simulink model "CtrPlatform"  (Simulink 7.9)
settings: Solver=ode3  StartTime=0.0  StopTime=8  FixedStep=Ts  RelTol=1e-3
InitFcn:
  | eval('CtrPlatformCfg')
StopFcn:
  | eval('CtrPlotTrj')
values from neighbouring files (symbols this model uses):
  A = [a1 a2 a3 a4 a5 a6]/180*pi    [Config.m]    (also in CtrPlatformCfg.m)
  a2 = 0    [Config.m]    (also in CtrPlatformCfg.m)
  a3 = 0    [Config.m]    (also in CtrPlatformCfg.m)
  a4 = 0    [Config.m]    (also in CtrPlatformCfg.m)
  a5 = 90    [Config.m]    (also in CtrPlatformCfg.m)
  a6 = 0    [Config.m]    (also in CtrPlatformCfg.m)
  Cen = Cen(:)'    [Config.m]    (also in CtrPlatformCfg.m; DynEulerTest.m = Cen'; EfDynCAD.m = [cen1,cen2,cen3,cen4,cen5,cen6]')
  CurPulseFreq = 0.25*2*pi    (= 1.57079632679)    [Config.m]    (also in CtrPlatformCfg.m)
  Deg2Rad = pi/180    (= 0.0174532925199)    [Config.m]    (also in CtrPlatformCfg.m)
  DisturbSelect = 2    [Config.m]    (also in CtrPlatformCfg.m)
  DynTrjMode = 3    [Config.m]    (also in CtrPlatformCfg.m = 1)
  FbDisturbSelect = 2    [Config.m]    (also in CtrPlatformCfg.m)
  freq = tvel/radius    (= 1)    [Config.m]    (also in CtrPlatformCfg.m)
  FrictionSelect = 2    [CtrPlatformCfg.m]
  Gravity = 9.8    [Config.m]    (also in CtrPlatformCfg.m)
  Ie1 = in1(:)'    [Config.m]    (also in CtrPlatformCfg.m; DynEulerTest.m = in1(:); EfDynCAD.m = in1(:))
  Ie2 = in2(:)'    [Config.m]    (also in CtrPlatformCfg.m; DynEulerTest.m = in2(:); EfDynCAD.m = in2(:))
  Ie3 = in3(:)'    [Config.m]    (also in CtrPlatformCfg.m; DynEulerTest.m = in3(:); EfDynCAD.m = in3(:))
  Ie4 = in4(:)'    [Config.m]    (also in CtrPlatformCfg.m; DynEulerTest.m = in4(:); EfDynCAD.m = in4(:))
  Ie5 = in5(:)'    [Config.m]    (also in CtrPlatformCfg.m; DynEulerTest.m = in5(:); EfDynCAD.m = in5(:))
  Ie6 = in6(:)'    [Config.m]    (also in CtrPlatformCfg.m; DynEulerTest.m = in6(:); EfDynCAD.m = in6(:))
  in1 = [5.2954 -0.2565 -0.6366;-0.2565 4.7000 0.2830;-0.6366 0.2829 5.8635]    [Config.m]    (also in CtrPlatformCfg.m; DynEulerTest.m; EfDynCAD.m = [0.54  -0.01 0.23)
  in2 = [5.8840 0.0072 0.0135;0.0072 6.0178 -0.1907;0.0135 -0.1907 0.3374]    [Config.m]    (also in CtrPlatformCfg.m; DynEulerTest.m; EfDynCAD.m = (R_x*R_z)*in2*(R_x*R_z)')
  in3 = [1.8201 -0.2274 -0.3112;-0.2274 2.2537 -0.1441;-0.3112 -0.1441 1.9485]    [Config.m]    (also in CtrPlatformCfg.m; DynEulerTest.m; EfDynCAD.m = (R_x*R_z)*in3*(R_x*R_z)')
  in4 = [0.0607 -0.0922 0;-0.0922 1.4493 0;0 0 1.4620]    [Config.m]    (also in CtrPlatformCfg.m; DynEulerTest.m = [0.0607 -0.0922 0;-0.0922 1.4493 0;0 0,1.4620]; EfDynCAD.m = (R_y*Rz)*in4*(R_y*Rz)')
  in5 = [0.0191 0.0032 0;0.0032 0.0228 0;0 0 0.0291]    [Config.m]    (also in CtrPlatformCfg.m; DynEulerTest.m; EfDynCAD.m = (R_x*R_y)*in5*(R_x*R_y)')
  in6 = [0.0012 0 0;0 0.0007 0;0 0 0.0007]    [Config.m]    (also in CtrPlatformCfg.m; DynEulerTest.m; EfDynCAD.m = (R_y*Rz)*in6*(R_y*Rz)')
  init_Endx = gd_init(1,4)    [Config.m]    (also in CtrPlatformCfg.m)
  init_Endy = gd_init(2,4)    [Config.m]    (also in CtrPlatformCfg.m)
  init_Endz = gd_init(3,4)    [Config.m]    (also in CtrPlatformCfg.m)
  init_Rot = gd_init(1:3,1:3)    [Config.m]    (also in CtrPlatformCfg.m)
  JntOffset1 = A(1)    [Config.m]    (also in CtrPlatformCfg.m)
  JntOffset2 = A(2)    [Config.m]    (also in CtrPlatformCfg.m)
  JntOffset3 = A(3)    [Config.m]    (also in CtrPlatformCfg.m)
  JntOffset4 = A(4)    [Config.m]    (also in CtrPlatformCfg.m)
  JntOffset5 = A(5)    [Config.m]    (also in CtrPlatformCfg.m)
  JntOffset6 = A(6)    [Config.m]    (also in CtrPlatformCfg.m)
  L = [l1 l2 l3 l4 l5 l6 l7 l8 l9]    [Config.m]    (also in CtrPlatformCfg.m)
  LinePTs2RadpS = 2*pi/(EncRes*Ts)./Gear    [Config.m]    (also in CtrPlatformCfg.m)
  LinePTs2Rpm = 60/(EncRes*Ts)    (= 7.32421875)    [Config.m]    (also in CtrPlatformCfg.m)
  Ma = [ma1 ma2 ma3 ma4 ma5 ma6]    [Config.m]    (also in CtrPlatformCfg.m; DynEulerTest.m = [ma1; ma2; ma3; ma4; ma5; ma6]; EfDynCAD.m = [ma1 ma2 ma3 ma4 ma5 ma6]')
  ma1 = 170.31    [Config.m]    (also in CtrPlatformCfg.m; DynEulerTest.m; EfDynCAD.m = 77.75)
  ma2 = 63.74    [Config.m]    (also in CtrPlatformCfg.m; DynEulerTest.m; EfDynCAD.m = 32.31)
  ma3 = 98.98    [Config.m]    (also in CtrPlatformCfg.m; DynEulerTest.m; EfDynCAD.m = 18.61)
  ma4 = 24.46    [Config.m]    (also in CtrPlatformCfg.m; DynEulerTest.m; EfDynCAD.m = 15.65)
  ma5 = 5.24    [Config.m]    (also in CtrPlatformCfg.m; DynEulerTest.m; EfDynCAD.m = 3.32)
  ma6 = 0.6    [Config.m]    (also in CtrPlatformCfg.m; DynEulerTest.m; EfDynCAD.m)
  PosPulseEnable = 1    [Config.m]    (also in CtrPlatformCfg.m)
  PosVelPulseGain = 500    [Config.m]    (also in CtrPlatformCfg.m)
  Rad2Line = Gear*EncRes/(2*pi)    [Config.m]    (also in CtrPlatformCfg.m)
  Rpm2LinePTs = EncRes*Ts/60    (= 0.136533333333)    [Config.m]    (also in CtrPlatformCfg.m)
  TrajSwitch = 1    [Config.m]    (also in CtrPlatformCfg.m)
  Trq2Cur = Trq2Cur./Cur2Trq    [Config.m]    (also in CtrPlatformCfg.m)
  Ts = 1/FrHz    (= 0.00025)    [Config.m]    (also in CtrPlatformCfg.m)
  Ts_Dyn = Ts    (= 0.00025)    [Config.m]    (also in CtrPlatformCfg.m)
  tvel = 120    [Config.m]    (also in CtrPlatformCfg.m)
  VelLpAxisNum = 1    [Config.m]    (also in CtrPlatformCfg.m)
  VelPulseEnable = 0    [Config.m]    (also in CtrPlatformCfg.m)
  VelPulseGain = 500    [Config.m]    (also in CtrPlatformCfg.m)
  Volt2Trq = Volt2Trq./Trq2Cur    [Config.m]    (also in CtrPlatformCfg.m)
undefined symbols (not defined in the file or in its folder): a1, DiscIntNeverNeededParam, RobotAxis
libraries: simulink x85, mblibv1 x35, powerlib_extras x25, commnoisgen2 x2
(part 1 of 5)
settings Model: Creator=DAI Dan  LastModifiedBy=Administrator
settings DebuggingCC: FcnCallInpInsideContextMsg=Use local settings
settings GRTTargetCC: CombineOutputUpdateFcns=off  GRTInterface=on
settings ConfigurationSet: Description=SimMechanics 2G

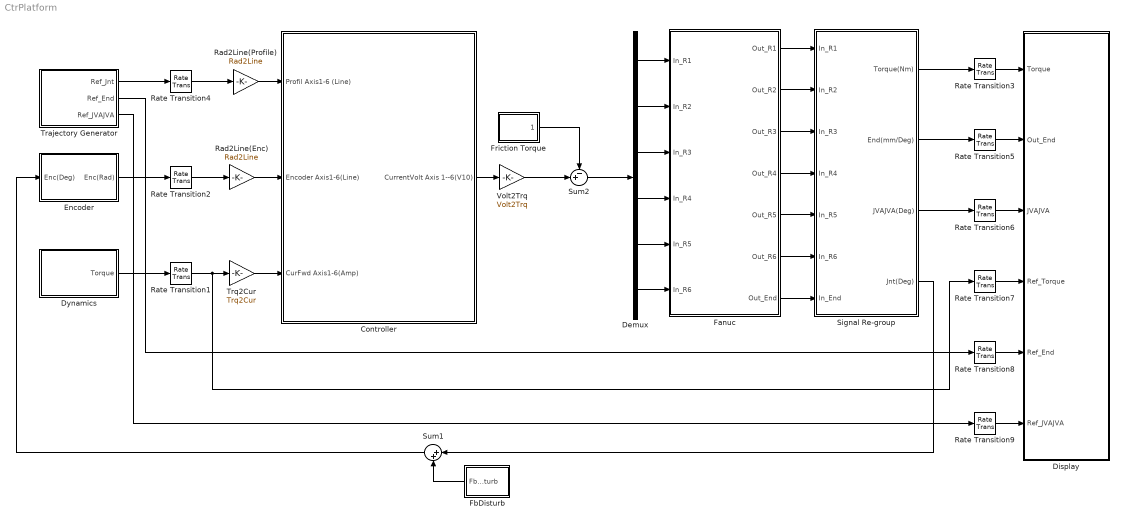
== system CtrPlatform ==
  Controller : Subsystem
  Demux : Demux  Outputs=6
  Display : Subsystem
  Dynamics : Subsystem
  Encoder : Subsystem
  Fanuc : Subsystem
  FbDisturb : Subsystem
  Friction Torque : Subsystem
  Rad2Line(Enc) : Gain  Gain=Rad2Line
  Rad2Line(Profile) : Gain  Gain=Rad2Line
  Rate Transition{1..9} (9 alike) : RateTransition  OutPortSampleTime=Ts
  Signal Re-group : Subsystem
  Sum1 : Sum  Inputs=|++
  Sum2 : Sum  Inputs=-+|
  Trajectory Generator : Subsystem
  Trq2Cur : Gain  Gain=Trq2Cur
  Volt2Trq : Gain  Gain=Volt2Trq  SampleTime=Ts
  wires:
  Trq2Cur/1 -> Controller/3(CurFwd Axis1-6(Amp))
  Rad2Line(Profile)/1 -> Controller/1(Profil Axis1-6 (Line))
  Rad2Line(Enc)/1 -> Controller/2(Encoder Axis1-6(Line))
  Controller/1(CurrentVolt Axis 1--6(V10)) -> Volt2Trq/1
  Rate Transition4/1 -> Rad2Line(Profile)/1
  Rate Transition1/1 -> Trq2Cur/1, Rate Transition7/1
  Rate Transition2/1 -> Rad2Line(Enc)/1
  FbDisturb/1(FbDisturb) -> Sum1/2
  Demux/1 -> Fanuc/1(In_R1)
  Demux/2 -> Fanuc/2(In_R2)
  Demux/3 -> Fanuc/3(In_R3)
  Demux/4 -> Fanuc/4(In_R4)
  Demux/5 -> Fanuc/5(In_R5)
  Demux/6 -> Fanuc/6(In_R6)
  Fanuc/1(Out_R1) -> Signal Re-group/1(In_R1)
  Fanuc/2(Out_R2) -> Signal Re-group/2(In_R2)
  Fanuc/3(Out_R3) -> Signal Re-group/3(In_R3)
  Fanuc/4(Out_R4) -> Signal Re-group/4(In_R4)
  Fanuc/5(Out_R5) -> Signal Re-group/5(In_R5)
  Fanuc/6(Out_R6) -> Signal Re-group/6(In_R6)
  Fanuc/7(Out_End) -> Signal Re-group/7(In_End)
  Signal Re-group/1(Torque(Nm)) -> Rate Transition3/1
  Signal Re-group/2(End(mm/Deg)) -> Rate Transition5/1
  Signal Re-group/3(JVAJVA(Deg)) -> Rate Transition6/1
  Rate Transition3/1 -> Display/1(Torque)
  Rate Transition5/1 -> Display/2(Out_End)
  Rate Transition6/1 -> Display/3(JVAJVA)
  Rate Transition7/1 -> Display/4(Ref_Torque)
  Rate Transition8/1 -> Display/5(Ref_End)
  Rate Transition9/1 -> Display/6(Ref_JVAJVA)
  Signal Re-group/4(Jnt(Deg)) -> Sum1/1
  Sum2/1 -> Demux/1
  Volt2Trq/1 -> Sum2/2
  Friction Torque/1(Friction) -> Sum2/1
  Trajectory Generator/1(Ref_Jnt) -> Rate Transition4/1
  Dynamics/1(Torque) -> Rate Transition1/1
  Encoder/1(Enc(Rad)) -> Rate Transition2/1
  Sum1/1 -> Encoder/1(Enc(Deg))
  Trajectory Generator/2(Ref_End) -> Rate Transition8/1
  Trajectory Generator/3(Ref_JVAJVA) -> Rate Transition9/1

== system CtrPlatform/Controller ==
  Profil Axis1-6 (Line) : Inport
  Encoder Axis1-6(Line) : Inport  Port=2
  CurFwd Axis1-6(Amp) : Inport  Port=3
  Chech Axis Error Flag : Logic  Inputs=6  AllPortsSameDT=off  OutDataTypeStr=boolean
  Controller Axis 1 : Subsystem  mask{RobotAxis=RobotAxis(1), Ts=Ts}
      mask prompts: RobotAxis "Robot Axis Controller Parameter"; Ts "Sample Time"
      mask init:
      | %% Source and Control Loop Selection
      | PosSourceSelect=RobotAxis.PosSourceSelect;
      | VelSourceSelect=RobotAxis.VelSourceSelect;
      | CurSourceSelect=RobotAxis.CurSourceSelect;
      | FilterSelect=RobotAxis.FilterSelect;
      | FwdSelect=RobotAxis.FwdSelect;
      | AxisNO=RobotAxis.AxisNO;
      | 
      | %% Controller Parameter
      | Kpp=RobotAxis.Kpp; % Kp for position loop
      | Kpi=RobotAxis.Kpi; 
      | Kpd=RobotAxis.Kpd;
      | VelLimit=RobotAxis.VelLimit;
      | 
      | Kvp=RobotAxis.Kvp; % Kp for velocity loop
      | Kvi=RobotAxis.Kvi;
      | Kvd=RobotAxis.Kvd;
      | CurLimit = RobotAxis.CurLimit;
      | 
      | Cur2Volt=RobotAxis.Cur2Volt;
      | 
      | %% Feedforward Param
      | VelFwdGain=RobotAxis.VelFwdGain;
      | CurFwdGain=RobotAxis.CurFwdGain;
      | 
      | %% Protection
      | VelErrorCheckLimit=RobotAxis.VelErrorCheckLimit;
      | PosErrorCheckLimit=RobotAxis.PosErrorCheckLimit;
      | 
      | %% Initial Positon (Line)
      | InitialPos=RobotAxis.InitialPos;
  Controller Axis 2 : Subsystem  mask{RobotAxis=RobotAxis(2), Ts=Ts}
      mask prompts: RobotAxis "Robot Axis Controller Parameter"; Ts "Sample Time"
      mask init: same as CtrPlatform/Controller/Controller Axis 1
  Controller Axis 3 : Subsystem  mask{RobotAxis=RobotAxis(3), Ts=Ts}
      mask prompts: RobotAxis "Robot Axis Controller Parameter"; Ts "Sample Time"
      mask init: same as CtrPlatform/Controller/Controller Axis 1
  Controller Axis 4 : Subsystem  mask{RobotAxis=RobotAxis(4), Ts=Ts}
      mask prompts: RobotAxis "Robot Axis Controller Parameter"; Ts "Sample Time"
      mask init: same as CtrPlatform/Controller/Controller Axis 1
  Controller Axis 5 : Subsystem  mask{RobotAxis=RobotAxis(5), Ts=Ts}
      mask prompts: RobotAxis "Robot Axis Controller Parameter"; Ts "Sample Time"
      mask init: same as CtrPlatform/Controller/Controller Axis 1
  Controller Axis 6 : Subsystem  mask{RobotAxis=RobotAxis(6), Ts=Ts}
      mask prompts: RobotAxis "Robot Axis Controller Parameter"; Ts "Sample Time"
      mask init: same as CtrPlatform/Controller/Controller Axis 1
  Disturb : Subsystem
  ErrDisplay : Scope
      settings: SaveName=ScopeData12
  Integer Delay : Delay  DelayLength=1  InitialCondition=A'.*Rad2Line  SampleTime=Ts
  Mux : Mux  Inputs=6
  Source Model : Subsystem
  Sum2 : Sum  Inputs=++|
  CurrentVolt Axis 1--6(V10) : Outport
  wires:
  Chech Axis Error Flag/1 -> ErrDisplay/1
  Profil Axis1-6 (Line)/1 -> Controller Axis 1/1(Prof), Controller Axis 2/1(Prof), Controller Axis 5/1(Prof), Controller Axis 6/1(Prof), Controller Axis 4/1(Prof), Controller Axis 3/1(Prof)
  Encoder Axis1-6(Line)/1 -> Integer Delay/1
  CurFwd Axis1-6(Amp)/1 -> Controller Axis 1/3(CurFwd), Controller Axis 2/3(CurFwd), Controller Axis 3/3(CurFwd), Controller Axis 5/3(CurFwd), Controller Axis 6/3(CurFwd), Controller Axis 4/3(CurFwd)
  Controller Axis 1/1(CurrentVolt(V10)) -> Mux/1  "Volt Axis1"
  Controller Axis 2/1(CurrentVolt(V10)) -> Mux/2
  Controller Axis 3/1(CurrentVolt(V10)) -> Mux/3
  Controller Axis 4/1(CurrentVolt(V10)) -> Mux/4
  Controller Axis 5/1(CurrentVolt(V10)) -> Mux/5
  Controller Axis 6/1(CurrentVolt(V10)) -> Mux/6
  Controller Axis 1/2(ErrFlag) -> Chech Axis Error Flag/1  "Error Axis1"
  Controller Axis 2/2(ErrFlag) -> Chech Axis Error Flag/2
  Controller Axis 3/2(ErrFlag) -> Chech Axis Error Flag/3
  Controller Axis 4/2(ErrFlag) -> Chech Axis Error Flag/4
  Controller Axis 5/2(ErrFlag) -> Chech Axis Error Flag/5
  Controller Axis 6/2(ErrFlag) -> Chech Axis Error Flag/6
  Integer Delay/1 -> Controller Axis 1/2(Enc), Controller Axis 2/2(Enc), Controller Axis 5/2(Enc), Controller Axis 6/2(Enc), Controller Axis 4/2(Enc), Controller Axis 3/2(Enc)
  Mux/1 -> Sum2/2
  Sum2/1 -> CurrentVolt Axis 1--6(V10)/1
  Disturb/1(Disturb) -> Sum2/1

== system CtrPlatform/Display ==
  Torque : Inport
  Out_End : Inport  Port=2
  JVAJVA : Inport  Port=3
  Ref_Torque : Inport  Port=4
  Ref_End : Inport  Port=5
  Ref_JVAJVA : Inport  Port=6
  EndTrjDisplay : Subsystem
  JntVelAccDisplay : Subsystem
  TorqueDisplay : Subsystem
  wires:
  Torque/1 -> TorqueDisplay/1(Torque)
  Ref_Torque/1 -> TorqueDisplay/2(Ref_Torque)
  JVAJVA/1 -> JntVelAccDisplay/1(JointVelAcc)
  Ref_JVAJVA/1 -> JntVelAccDisplay/2(Ref_JntVelAcc)
  Out_End/1 -> EndTrjDisplay/1(End)
  Ref_End/1 -> EndTrjDisplay/2(RefEnd)

== system CtrPlatform/Dynamics ==
  C*Omega : MATLAB Function  TreatAsAtomicUnit=on
  C_Omega Display : Subsystem
  M*Acc : MATLAB Function  TreatAsAtomicUnit=on
  M_Acc Display : Subsystem
  N : MATLAB Function  TreatAsAtomicUnit=on
  N Display : Subsystem
  Rate Transition1 : RateTransition  OutPortSampleTime=Ts_Dyn
  Rate Transition2 : RateTransition  OutPortSampleTime=Ts_Dyn
  Rate Transition3 : RateTransition  OutPortSampleTime=Ts_Dyn
  Sum : Sum  Inputs=+++
  Terminator : Terminator
  Terminator1 : Terminator
  Terminator2 : Terminator
  Torque Display : Subsystem
  TrjSource : Subsystem
  Torque : Outport
  wires:
  M*Acc/1(M_Acc) -> Sum/1, M_Acc Display/1(M_Acc)
  C*Omega/1(C_Omega) -> Sum/3, C_Omega Display/1(C_Omega)
  Sum/1 -> Torque/1, Torque Display/1(Torque)
  N/1(N) -> Sum/2, N Display/1(N)
  [RobotEncPos] -> Rate Transition1/1
  [RobotEncVel] -> Rate Transition2/1
  [RobotEncAcc] -> Rate Transition3/1
  Rate Transition1/1 -> Terminator/1
  Rate Transition2/1 -> Terminator1/1
  Rate Transition3/1 -> Terminator2/1
  TrjSource/1(RefJntPos(Rad)) -> M*Acc/2(EnTheta), N/1(EnTheta), C*Omega/2(EnTheta)
  TrjSource/2(RefJntVel(Rad/s)) -> C*Omega/1(RefOmega), C*Omega/3(EnOmega)
  TrjSource/3(RefJntAcc(Rad/s2)) -> M*Acc/1(RefAcc)

== system CtrPlatform/Encoder ==
  Enc(Deg) : Inport
  Deg2Rad : Gain  Gain=Deg2Rad
  Demux1 : Demux  Outputs=6
  Dir{1..6} (6 alike) : Gain
  Mux : Mux  Inputs=6
  Enc(Rad) : Outport
  wires:
  Enc(Deg)/1 -> Deg2Rad/1
  Dir1/1 -> Mux/1
  Mux/1 -> Enc(Rad)/1
  Deg2Rad/1 -> Demux1/1
  Dir2/1 -> Mux/2
  Dir3/1 -> Mux/3
  Demux1/6 -> Dir6/1
  Dir6/1 -> Mux/6
  Dir5/1 -> Mux/5
  Dir4/1 -> Mux/4
  Demux1/5 -> Dir5/1
  Demux1/4 -> Dir4/1
  Demux1/3 -> Dir3/1
  Demux1/2 -> Dir2/1
  Demux1/1 -> Dir1/1

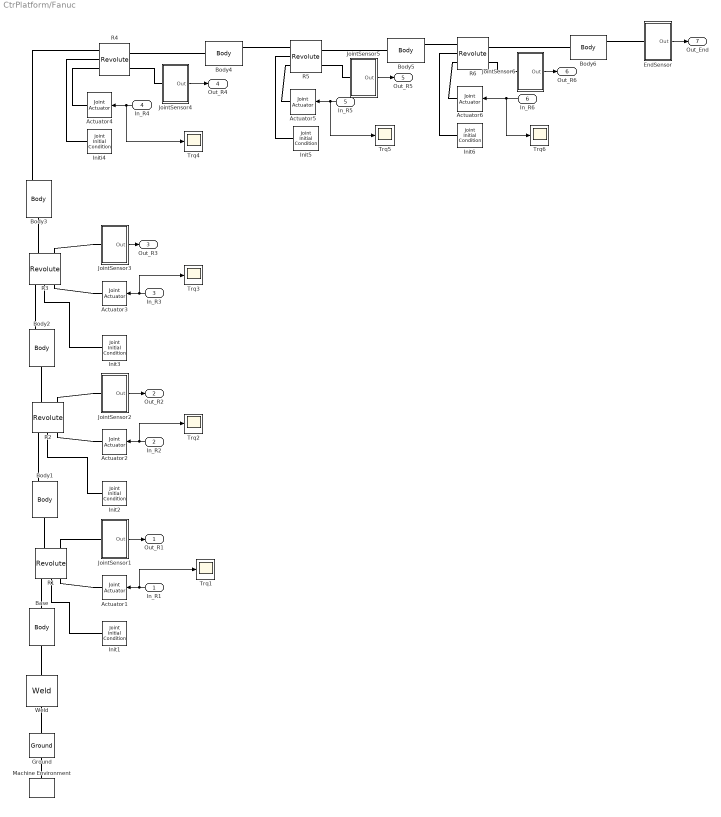
== system CtrPlatform/Fanuc ==
  In_R1 : Inport
  In_R2 : Inport  Port=2
  In_R3 : Inport  Port=3
  In_R4 : Inport  Port=4
  In_R5 : Inport  Port=5
  In_R6 : Inport  Port=6
  " EndSensor" : Subsystem
  Actuator{1..6} (6 alike) : mblibv1/Sensors &  Actuators/Joint Actuator  UpdateFromCAD=off  PhysicalDomain=Mechanical  PortType=blob  ActuationStyle=Force  AngleUnits=rad  ArcVelocityUnits=rad/s  ArcAccelerationUnits=rad/s^2  CoordPositionUnits=m  VelocityUnits=m/s  AccelerationUnits=m/s^2  ForceUnits=N  TorqueUnits=N*m  ActiveIO=on  Width=1  DialogClass=MechanicalActuatorBlock  Primitive=R1  ReferenceFrame=Absolute (World)
  Base : mblibv1/Bodies/Body  LConnTagsString=CS1  RConnTagsString=CS2  UpdateFromCAD=on  DialogClass=MechanicalBodyBlock  Mass=133.95  MassUnits=kg  InertiaUnits=kg*m^2  Inertia=[3.0977 0.0155 -0.0939;0.0155 3.3580 0.0061;-0.0939 0.0061 5.1969]  Shape=Cylinder  ShapeDims=[1 1]  ShapeUnits=m  ShapeUse=false  Density=1  DensityUnits=kg/m^3  DensityUse=false  GraphicsMode=GFXFILE  GraphicsFileName=M-710iC50 M-710iC70 - M-710iC50 M-710iC70 base-1.STL  BodyColorSelMode=COLORPALETTE  BodyColor=[0.25098 0.25098 0.25098]  AttachedToCS=CS1  CG=Right$CG$[-0.0437 -0.0026 0.1059]$WORLD$WORLD$m$[1 0 0;0 1 0;0 0 1]$3x3 Transform$rad$WORLD$false$none  WorkingFrames=Left$CS1$[0 0 0]$WORLD$WORLD$m$[1 0 0;0 1 0;0 0 1]$3x3 Transform$rad$WORLD$true$none#Right$CS2$[0 0 0.266]$WORLD$WORLD$m$[1 0 0;0 1 0;0 0 1]$3x3 Transform$rad$WORLD$true$none  CGPos=[-0.0437 -0.0026 0.1059]  CGRot=[1 0 0;0 1 0;0 0 1]  CS0Pos=[]  CS0Rot=[]  CS1Pos=[0 0 0]  CS1Rot=[1 0 0;0 1 0;0 0 1]  CS2Pos=[0 0 0.266]  CS2Rot=[1 0 0;0 1 0;0 0 1]  CS3Pos=[]  CS3Rot=[]  CS4Pos=[]  CS4Rot=[]  CS5Pos=[]  CS5Rot=[]  CS6Pos=[]  CS6Rot=[]  CS7Pos=[]  CS7Rot=[]  CS8Pos=[]  CS8Rot=[]  CS9Pos=[]  CS9Rot=[]  CS10Pos=[]  CS10Rot=[]  CS11Pos=[]  CS11Rot=[]  CS12Pos=[]  CS12Rot=[]  CS13Pos=[]  CS13Rot=[]  CS14Pos=[]  CS14Rot=[]  CS15Pos=[]  CS15Rot=[]  CS16Pos=[]  CS16Rot=[]  CS17Pos=[]  CS17Rot=[]  CS18Pos=[]  CS18Rot=[]  CS19Pos=[]  CS19Rot=[]  CS20Pos=[]  CS20Rot=[]
  Body1 : mblibv1/Bodies/Body  LConnTagsString=CS2  RConnTagsString=CS3|CS4  UpdateFromCAD=on  DialogClass=MechanicalBodyBlock  Mass=ma1  MassUnits=kg  InertiaUnits=kg*m^2  Inertia=in1  Shape=Cylinder  ShapeDims=[1 1]  ShapeUnits=m  ShapeUse=false  Density=1  DensityUnits=kg/m^3  DensityUse=false  GraphicsMode=GFXFILE  GraphicsFileName=M-710iC50 M-710iC70 - M-710iC50 M-710iC70 axis1-1.STL  BodyColorSelMode=COLORPALETTE  BodyColor=[0.86667 0.86667 0.8902]  AttachedToCS=CS1  CG=Right$CG$cen1$WORLD$WORLD$m$[1 0 0;0 1 0;0 0 1]$3x3 Transform$rad$WORLD$false$none  WorkingFrames=Right$CS1$cen1_1$WORLD$WORLD$m$[1 0 0;0 1 0;0 0 1]$3x3 Transform$rad$WORLD$false$none#Left$CS2$cen1_2$WORLD$WORLD$m$[1 0 0;0 1 0;0 0 1]$3x3 Transform$rad$WORLD$true$none#Right$CS3$cen1_3$WORLD$WORLD$m$[1 0 0;0 1 0;0 0 1]$3x3 Transform$rad$WORLD$true$none#Right$CS4$cen1_4$WORLD$WORLD$m$[1 0 0;0 1 0;0 0 1]$3x3 Transform$rad$WORLD$true$none  CGPos=cen1  CGRot=[1 0 0;0 1 0;0 0 1]  CS0Pos=[]  CS0Rot=[]  CS1Pos=cen1_1  CS1Rot=[1 0 0;0 1 0;0 0 1]  CS2Pos=cen1_2  CS2Rot=[1 0 0;0 1 0;0 0 1]  CS3Pos=cen1_3  CS3Rot=[1 0 0;0 1 0;0 0 1]  CS4Pos=cen1_4  CS4Rot=[1 0 0;0 1 0;0 0 1]  CS5Pos=[]  CS5Rot=[]  CS6Pos=[]  CS6Rot=[]  CS7Pos=[]  CS7Rot=[]  CS8Pos=[]  CS8Rot=[]  CS9Pos=[]  CS9Rot=[]  CS10Pos=[]  CS10Rot=[]  CS11Pos=[]  CS11Rot=[]  CS12Pos=[]  CS12Rot=[]  CS13Pos=[]  CS13Rot=[]  CS14Pos=[]  CS14Rot=[]  CS15Pos=[]  CS15Rot=[]  CS16Pos=[]  CS16Rot=[]  CS17Pos=[]  CS17Rot=[]  CS18Pos=[]  CS18Rot=[]  CS19Pos=[]  CS19Rot=[]  CS20Pos=[]  CS20Rot=[]
  Body2 : mblibv1/Bodies/Body  LConnTagsString=CS2  RConnTagsString=CS3|CS4  UpdateFromCAD=on  DialogClass=MechanicalBodyBlock  Mass=ma2  MassUnits=kg  InertiaUnits=kg*m^2  Inertia=in2  Shape=Cylinder  ShapeDims=[1 1]  ShapeUnits=m  ShapeUse=false  Density=1  DensityUnits=kg/m^3  DensityUse=false  GraphicsMode=GFXFILE  GraphicsFileName=M-710iC50 M-710iC70 - M-710iC50 M-710iC70 axis2-1.STL  BodyColorSelMode=COLORPALETTE  BodyColor=[1 1 0]  AttachedToCS=CS1  CG=Right$CG$cen2$WORLD$WORLD$m$[1 0 0;0 1 0;0 0 1]$3x3 Transform$rad$WORLD$false$none  WorkingFrames=Right$CS1$cen2_1$WORLD$WORLD$m$[1 0 0;0 1 0;0 0 1]$3x3 Transform$rad$WORLD$false$none#Left$CS2$cen2_2$WORLD$WORLD$m$[1 0 0;0 1 0;0 0 1]$3x3 Transform$rad$WORLD$true$none#Right$CS3$cen2_3$WORLD$WORLD$m$[1 0 0;0 1 0;0 0 1]$3x3 Transform$rad$WORLD$true$none#Right$CS4$cen2_4$WORLD$WORLD$m$[1 0 0;0 1 0;0 0 1]$3x3 Transform$rad$WORLD$true$none  CGPos=cen2  CGRot=[1 0 0;0 1 0;0 0 1]  CS0Pos=[]  CS0Rot=[]  CS1Pos=cen2_1  CS1Rot=[1 0 0;0 1 0;0 0 1]  CS2Pos=cen2_2  CS2Rot=[1 0 0;0 1 0;0 0 1]  CS3Pos=cen2_3  CS3Rot=[1 0 0;0 1 0;0 0 1]  CS4Pos=cen2_4  CS4Rot=[1 0 0;0 1 0;0 0 1]  CS5Pos=[]  CS5Rot=[]  CS6Pos=[]  CS6Rot=[]  CS7Pos=[]  CS7Rot=[]  CS8Pos=[]  CS8Rot=[]  CS9Pos=[]  CS9Rot=[]  CS10Pos=[]  CS10Rot=[]  CS11Pos=[]  CS11Rot=[]  CS12Pos=[]  CS12Rot=[]  CS13Pos=[]  CS13Rot=[]  CS14Pos=[]  CS14Rot=[]  CS15Pos=[]  CS15Rot=[]  CS16Pos=[]  CS16Rot=[]  CS17Pos=[]  CS17Rot=[]  CS18Pos=[]  CS18Rot=[]  CS19Pos=[]  CS19Rot=[]  CS20Pos=[]  CS20Rot=[]
  Body3 : mblibv1/Bodies/Body  LConnTagsString=CS2  RConnTagsString=CS3|CS4  UpdateFromCAD=on  DialogClass=MechanicalBodyBlock  Mass=ma3  MassUnits=kg  InertiaUnits=kg*m^2  Inertia=in3  Shape=Cylinder  ShapeDims=[1 1]  ShapeUnits=m  ShapeUse=false  Density=1  DensityUnits=kg/m^3  DensityUse=false  GraphicsMode=GFXFILE  GraphicsFileName=M-710iC50 M-710iC70 - M-710iC50 M-710iC70 axis3-1.STL  BodyColorSelMode=COLORPALETTE  BodyColor=[1 1 0]  AttachedToCS=CS1  CG=Right$CG$cen3$WORLD$WORLD$m$[1 0 0;0 1 0;0 0 1]$3x3 Transform$rad$WORLD$false$none  WorkingFrames=Right$CS1$cen3_1$WORLD$WORLD$m$[1 0 0;0 1 0;0 0 1]$3x3 Transform$rad$WORLD$false$none#Left$CS2$cen3_2$WORLD$WORLD$m$[1 0 0;0 1 0;0 0 1]$3x3 Transform$rad$WORLD$true$none#Right$CS3$cen3_3$WORLD$WORLD$m$[1 0 0;0 1 0;0 0 1]$3x3 Transform$rad$WORLD$true$none#Right$CS4$cen3_4$WORLD$WORLD$m$[1 0 0;0 1 0;0 0 1]$3x3 Transform$rad$WORLD$true$none  CGPos=cen3  CGRot=[1 0 0;0 1 0;0 0 1]  CS0Pos=[]  CS0Rot=[]  CS1Pos=cen3_1  CS1Rot=[1 0 0;0 1 0;0 0 1]  CS2Pos=cen3_2  CS2Rot=[1 0 0;0 1 0;0 0 1]  CS3Pos=cen3_3  CS3Rot=[1 0 0;0 1 0;0 0 1]  CS4Pos=cen3_4  CS4Rot=[1 0 0;0 1 0;0 0 1]  CS5Pos=[]  CS5Rot=[]  CS6Pos=[]  CS6Rot=[]  CS7Pos=[]  CS7Rot=[]  CS8Pos=[]  CS8Rot=[]  CS9Pos=[]  CS9Rot=[]  CS10Pos=[]  CS10Rot=[]  CS11Pos=[]  CS11Rot=[]  CS12Pos=[]  CS12Rot=[]  CS13Pos=[]  CS13Rot=[]  CS14Pos=[]  CS14Rot=[]  CS15Pos=[]  CS15Rot=[]  CS16Pos=[]  CS16Rot=[]  CS17Pos=[]  CS17Rot=[]  CS18Pos=[]  CS18Rot=[]  CS19Pos=[]  CS19Rot=[]  CS20Pos=[]  CS20Rot=[]
  Body4 : mblibv1/Bodies/Body  LConnTagsString=CS2  RConnTagsString=CS3|CS4  UpdateFromCAD=on  DialogClass=MechanicalBodyBlock  Mass=ma4  MassUnits=kg  InertiaUnits=kg*m^2  Inertia=in4  Shape=Cylinder  ShapeDims=[1 1]  ShapeUnits=m  ShapeUse=false  Density=1  DensityUnits=kg/m^3  DensityUse=false  GraphicsMode=GFXFILE  GraphicsFileName=M-710iC50 M-710iC70 - M-710iC50 M-710iC70 axis4-1.STL  BodyColorSelMode=COLORPALETTE  BodyColor=[1 1 0]  AttachedToCS=CS1  CG=Right$CG$cen4$WORLD$WORLD$m$[1 0 0;0 0 1;0 -1 0]$3x3 Transform$rad$WORLD$false$none  WorkingFrames=Right$CS1$cen4_1$WORLD$WORLD$m$[1 0 0;0 0 1;0 -1 0]$3x3 Transform$rad$WORLD$false$none#Left$CS2$cen4_2$WORLD$WORLD$m$[1 0 0;0 1 0;0 0 1]$3x3 Transform$rad$WORLD$true$none#Right$CS3$cen4_3$WORLD$WORLD$m$[1 0 0;0 1 0;0 0 1]$3x3 Transform$rad$WORLD$true$none#Right$CS4$cen4_4$WORLD$WORLD$m$[1 0 0;0 1 0;0 0 1]$3x3 Transform$rad$WORLD$true$none  CGPos=cen4  CGRot=[1 0 0;0 0 1;0 -1 0]  CS0Pos=[]  CS0Rot=[]  CS1Pos=cen4_1  CS1Rot=[1 0 0;0 0 1;0 -1 0]  CS2Pos=cen4_2  CS2Rot=[1 0 0;0 1 0;0 0 1]  CS3Pos=cen4_3  CS3Rot=[1 0 0;0 1 0;0 0 1]  CS4Pos=cen4_4  CS4Rot=[1 0 0;0 1 0;0 0 1]  CS5Pos=[]  CS5Rot=[]  CS6Pos=[]  CS6Rot=[]  CS7Pos=[]  CS7Rot=[]  CS8Pos=[]  CS8Rot=[]  CS9Pos=[]  CS9Rot=[]  CS10Pos=[]  CS10Rot=[]  CS11Pos=[]  CS11Rot=[]  CS12Pos=[]  CS12Rot=[]  CS13Pos=[]  CS13Rot=[]  CS14Pos=[]  CS14Rot=[]  CS15Pos=[]  CS15Rot=[]  CS16Pos=[]  CS16Rot=[]  CS17Pos=[]  CS17Rot=[]  CS18Pos=[]  CS18Rot=[]  CS19Pos=[]  CS19Rot=[]  CS20Pos=[]  CS20Rot=[]
  Body5 : mblibv1/Bodies/Body  LConnTagsString=CS2  RConnTagsString=CS3|CS4  UpdateFromCAD=on  DialogClass=MechanicalBodyBlock  Mass=ma5  MassUnits=kg  InertiaUnits=kg*m^2  Inertia=in5  Shape=Cylinder  ShapeDims=[1 1]  ShapeUnits=m  ShapeUse=false  Density=1  DensityUnits=kg/m^3  DensityUse=false  GraphicsMode=GFXFILE  GraphicsFileName=M-710iC50 M-710iC70 - M-710iC50 M-710iC70 axis5-1.STL  BodyColorSelMode=COLORPALETTE  BodyColor=[1 1 0]  AttachedToCS=CS1  CG=Right$CG$cen5$WORLD$WORLD$m$[1 0 0;0 1 0;0 0 1]$3x3 Transform$rad$WORLD$false$none  WorkingFrames=Right$CS1$cen5_1$WORLD$WORLD$m$[1 0 0;0 1 0;0 0 1]$3x3 Transform$rad$WORLD$false$none#Left$CS2$cen5_2$WORLD$WORLD$m$[1 0 0;0 1 0;0 0 1]$3x3 Transform$rad$WORLD$true$none#Right$CS3$cen5_3$WORLD$WORLD$m$[1 0 0;0 1 0;0 0 1]$3x3 Transform$rad$WORLD$true$none#Right$CS4$cen5_4$WORLD$WORLD$m$[1 0 0;0 1 0;0 0 1]$3x3 Transform$rad$WORLD$true$none  CGPos=cen5  CGRot=[1 0 0;0 1 0;0 0 1]  CS0Pos=[]  CS0Rot=[]  CS1Pos=cen5_1  CS1Rot=[1 0 0;0 1 0;0 0 1]  CS2Pos=cen5_2  CS2Rot=[1 0 0;0 1 0;0 0 1]  CS3Pos=cen5_3  CS3Rot=[1 0 0;0 1 0;0 0 1]  CS4Pos=cen5_4  CS4Rot=[1 0 0;0 1 0;0 0 1]  CS5Pos=[]  CS5Rot=[]  CS6Pos=[]  CS6Rot=[]  CS7Pos=[]  CS7Rot=[]  CS8Pos=[]  CS8Rot=[]  CS9Pos=[]  CS9Rot=[]  CS10Pos=[]  CS10Rot=[]  CS11Pos=[]  CS11Rot=[]  CS12Pos=[]  CS12Rot=[]  CS13Pos=[]  CS13Rot=[]  CS14Pos=[]  CS14Rot=[]  CS15Pos=[]  CS15Rot=[]  CS16Pos=[]  CS16Rot=[]  CS17Pos=[]  CS17Rot=[]  CS18Pos=[]  CS18Rot=[]  CS19Pos=[]  CS19Rot=[]  CS20Pos=[]  CS20Rot=[]
  Body6 : mblibv1/Bodies/Body  LConnTagsString=CS2  RConnTagsString=CS3|CS4  UpdateFromCAD=on  DialogClass=MechanicalBodyBlock  Mass=ma6  MassUnits=kg  InertiaUnits=kg*m^2  Inertia=in6  Shape=Cylinder  ShapeDims=[1 1]  ShapeUnits=m  ShapeUse=false  Density=1  DensityUnits=kg/m^3  DensityUse=false  GraphicsMode=GFXFILE  GraphicsFileName=M-710iC50 M-710iC70 - M-710iC50 M-710iC70 axis6-1.STL  BodyColorSelMode=COLORPALETTE  BodyColor=[0.75294 0.75294 0.75294]  AttachedToCS=CS1  CG=Right$CG$cen6$WORLD$WORLD$m$[1 0 0;0 1 0;0 0 1]$3x3 Transform$rad$WORLD$false$none  WorkingFrames=Right$CS1$cen6_1$WORLD$WORLD$m$[0 0 1;0 -1 0;1 0 0]$3x3 Transform$rad$WORLD$false$none#Left$CS2$cen6_2$WORLD$WORLD$m$[1 0 0;0 1 0;0 0 1]$3x3 Transform$rad$WORLD$true$none#Right$CS3$cen6_3$WORLD$WORLD$m$[1 0 0;0 1 0;0 0 1]$3x3 Transform$rad$WORLD$true$none#Right$CS4$cen6_4$WORLD$WORLD$m$[1 0 0;0 1 0;0 0 1]$3x3 Transform$rad$WORLD$true$none  CGPos=cen6  CGRot=[1 0 0;0 1 0;0 0 1]  CS0Pos=[]  CS0Rot=[]  CS1Pos=cen6_1  CS1Rot=[0 0 1;0 -1 0;1 0 0]  CS2Pos=cen6_2  CS2Rot=[1 0 0;0 1 0;0 0 1]  CS3Pos=cen6_3  CS3Rot=[1 0 0;0 1 0;0 0 1]  CS4Pos=cen6_4  CS4Rot=[1 0 0;0 1 0;0 0 1]  CS5Pos=[]  CS5Rot=[]  CS6Pos=[]  CS6Rot=[]  CS7Pos=[]  CS7Rot=[]  CS8Pos=[]  CS8Rot=[]  CS9Pos=[]  CS9Rot=[]  CS10Pos=[]  CS10Rot=[]  CS11Pos=[]  CS11Rot=[]  CS12Pos=[]  CS12Rot=[]  CS13Pos=[]  CS13Rot=[]  CS14Pos=[]  CS14Rot=[]  CS15Pos=[]  CS15Rot=[]  CS16Pos=[]  CS16Rot=[]  CS17Pos=[]  CS17Rot=[]  CS18Pos=[]  CS18Rot=[]  CS19Pos=[]  CS19Rot=[]  CS20Pos=[]  CS20Rot=[]
  Ground : mblibv1/Bodies/Ground  UpdateFromCAD=on  LeftPortType=env  RightPortType=workingframe  PhysicalDomain=Mechanical  DialogClass=GroundBlock  CoordPosition=[0 0 0]  CoordPositionUnits=m  StateVectorMgrId=-1  MachineId=[0 0]  ShowEnvPort=on
      link override _mech_engine/ToBlock2: GotoTag=sim_mech_tag8d75a0291950a803
  Init1 : mblibv1/Sensors &  Actuators/Joint Initial Condition  UpdateFromCAD=off  LeftPortType=blob  RightPortType=blob  PhysicalDomain=mechanical  DialogClass=InitialConditionBlock  InitialConditions=P1$false$0$m$deg$0$m/s$deg/s#P2$false$0$m$deg$0$m/s$deg/s#P3$false$0$m$deg$0$m/s$deg/s#R1$true$a1$m$deg$0$m/s$deg/s#R2$false$0$m$deg$0$m/s$deg/s#R3$false$0$m$deg$0$m/s$deg/s#S$false$0$m$deg$0$m/s$deg/s  P1PIC=0  P1VIC=0  P2PIC=0  P2VIC=0  P3PIC=0  P3VIC=0  R1PIC=a1  R1VIC=0  R2PIC=0  R2VIC=0  R3PIC=0  R3VIC=0  SPIC=0  SVIC=0
  Init2 : mblibv1/Sensors &  Actuators/Joint Initial Condition  UpdateFromCAD=off  LeftPortType=blob  RightPortType=blob  PhysicalDomain=mechanical  DialogClass=InitialConditionBlock  InitialConditions=P1$false$0$m$deg$0$m/s$deg/s#P2$false$0$m$deg$0$m/s$deg/s#P3$false$0$m$deg$0$m/s$deg/s#R1$true$a2$m$deg$0$m/s$deg/s#R2$false$0$m$deg$0$m/s$deg/s#R3$false$0$m$deg$0$m/s$deg/s#S$false$0$m$deg$0$m/s$deg/s  P1PIC=0  P1VIC=0  P2PIC=0  P2VIC=0  P3PIC=0  P3VIC=0  R1PIC=a2  R1VIC=0  R2PIC=0  R2VIC=0  R3PIC=0  R3VIC=0  SPIC=0  SVIC=0
  Init3 : mblibv1/Sensors &  Actuators/Joint Initial Condition  UpdateFromCAD=off  LeftPortType=blob  RightPortType=blob  PhysicalDomain=mechanical  DialogClass=InitialConditionBlock  InitialConditions=P1$false$0$m$deg$0$m/s$deg/s#P2$false$0$m$deg$0$m/s$deg/s#P3$false$0$m$deg$0$m/s$deg/s#R1$true$a3$m$deg$0$m/s$deg/s#R2$false$0$m$deg$0$m/s$deg/s#R3$false$0$m$deg$0$m/s$deg/s#S$false$0$m$deg$0$m/s$deg/s  P1PIC=0  P1VIC=0  P2PIC=0  P2VIC=0  P3PIC=0  P3VIC=0  R1PIC=a3  R1VIC=0  R2PIC=0  R2VIC=0  R3PIC=0  R3VIC=0  SPIC=0  SVIC=0
  Init5 : mblibv1/Sensors &  Actuators/Joint Initial Condition  UpdateFromCAD=off  LeftPortType=blob  RightPortType=blob  PhysicalDomain=mechanical  DialogClass=InitialConditionBlock  InitialConditions=P1$false$0$m$deg$0$m/s$deg/s#P2$false$0$m$deg$0$m/s$deg/s#P3$false$0$m$deg$0$m/s$deg/s#R1$true$a5$m$deg$0$m/s$deg/s#R2$false$0$m$deg$0$m/s$deg/s#R3$false$0$m$deg$0$m/s$deg/s#S$false$0$m$deg$0$m/s$deg/s  P1PIC=0  P1VIC=0  P2PIC=0  P2VIC=0  P3PIC=0  P3VIC=0  R1PIC=a5  R1VIC=0  R2PIC=0  R2VIC=0  R3PIC=0  R3VIC=0  SPIC=0  SVIC=0
  Init6 : mblibv1/Sensors &  Actuators/Joint Initial Condition  UpdateFromCAD=off  LeftPortType=blob  RightPortType=blob  PhysicalDomain=mechanical  DialogClass=InitialConditionBlock  InitialConditions=P1$false$0$m$deg$0$m/s$deg/s#P2$false$0$m$deg$0$m/s$deg/s#P3$false$0$m$deg$0$m/s$deg/s#R1$true$a6$m$deg$0$m/s$deg/s#R2$false$0$m$deg$0$m/s$deg/s#R3$false$0$m$deg$0$m/s$deg/s#S$false$0$m$deg$0$m/s$deg/s  P1PIC=0  P1VIC=0  P2PIC=0  P2VIC=0  P3PIC=0  P3VIC=0  R1PIC=a6  R1VIC=0  R2PIC=0  R2VIC=0  R3PIC=0  R3VIC=0  SPIC=0  SVIC=0
  Initi4 : mblibv1/Sensors &  Actuators/Joint Initial Condition  UpdateFromCAD=off  LeftPortType=blob  RightPortType=blob  PhysicalDomain=mechanical  DialogClass=InitialConditionBlock  InitialConditions=P1$false$0$m$deg$0$m/s$deg/s#P2$false$0$m$deg$0$m/s$deg/s#P3$false$0$m$deg$0$m/s$deg/s#R1$true$a4$m$deg$0$m/s$deg/s#R2$false$0$m$deg$0$m/s$deg/s#R3$false$0$m$deg$0$m/s$deg/s#S$false$0$m$deg$0$m/s$deg/s  P1PIC=0  P1VIC=0  P2PIC=0  P2VIC=0  P3PIC=0  P3VIC=0  R1PIC=a4  R1VIC=0  R2PIC=0  R2VIC=0  R3PIC=0  R3VIC=0  SPIC=0  SVIC=0
  JointSensor1 : Subsystem
  JointSensor2 : Subsystem
  JointSensor3 : Subsystem
  JointSensor4 : Subsystem
  JointSensor5 : Subsystem
  JointSensor6 : Subsystem
  Machine Environment : mblibv1/Bodies/Machine Environment  PortType=env  PhysicalDomain=Mechanical  DialogTemplateClass=MECH.MachineEnvironment  SyncWhenCopied=off  Gravity=[0 0 -Gravity]  GravityUnits=m/s^2  GravityAsSignal=off  Dimensionality=Auto-detect  AnalysisType=Forward dynamics  LinearAssemblyTolerance=1e-3  LinearAssemblyToleranceUnits=m  AngularAssemblyTolerance=1e-3  AngularAssemblyToleranceUnits=rad  ConstraintSolverType=Stabilizing  ConstraintRelTolerance=1e-4  ConstraintAbsTolerance=1e-4  UseRobustSingularityHandling=off  RedundancyAnalysisToleranceType=Automatically select tolerance  RedundancyAnalysisTolerance=1e-14  StatePerturbationType=Fixed  PerturbationSize=1e-5  VisualizeMachine=on  BodyVisualizationType=Use model default body geometries  BodyColorSelMode=Use model default  DefaultBodyColor=[1 0 0]
  R1 : mblibv1/Joints/Revolute  LConnTagsString=__newl0|SA1|SA2  RConnTagsString=__newr0|SA1  UpdateFromCAD=on  NumSAPorts=3  CutJoint=off  MarkAsCut=off  Primitives=prismatic  PrimitiveProps=R1$World$[0,0,1]$revolute  DialogClass=JointBlock  R1Axis=[0,0,1]
  R2 : mblibv1/Joints/Revolute  LConnTagsString=__newl0|SA1|SA2  RConnTagsString=__newr0|SA1  UpdateFromCAD=on  NumSAPorts=3  CutJoint=off  MarkAsCut=off  Primitives=prismatic  PrimitiveProps=R1$World$[0,1,0]$revolute  DialogClass=JointBlock  R1Axis=[0,1,0]
  R3 : mblibv1/Joints/Revolute  LConnTagsString=__newl0|SA1|SA2  RConnTagsString=__newr0|SA1  UpdateFromCAD=on  NumSAPorts=3  CutJoint=off  MarkAsCut=off  Primitives=prismatic  PrimitiveProps=R1$World$[0,1,0]$revolute  DialogClass=JointBlock  R1Axis=[0,1,0]
  R4 : mblibv1/Joints/Revolute  LConnTagsString=__newl0|SA1|SA2  RConnTagsString=__newr0|SA1  UpdateFromCAD=on  NumSAPorts=3  CutJoint=off  MarkAsCut=off  Primitives=prismatic  PrimitiveProps=R1$World$[1,0,0]$revolute  DialogClass=JointBlock  R1Axis=[1,0,0]
  R5 : mblibv1/Joints/Revolute  LConnTagsString=__newl0|SA1|SA2  RConnTagsString=__newr0|SA1  UpdateFromCAD=on  NumSAPorts=3  CutJoint=off  MarkAsCut=off  Primitives=prismatic  PrimitiveProps=R1$World$[0,1,0]$revolute  DialogClass=JointBlock  R1Axis=[0,1,0]
  R6 : mblibv1/Joints/Revolute  LConnTagsString=__newl0|SA1|SA2  RConnTagsString=__newr0|SA1  UpdateFromCAD=on  NumSAPorts=3  CutJoint=off  MarkAsCut=off  Primitives=prismatic  PrimitiveProps=R1$World$[1,0,0]$revolute  DialogClass=JointBlock  R1Axis=[1,0,0]
  Trq{1..6} (6 alike) : Scope
      Trq1 settings: SaveName=ScopeData13
      Trq2 settings: SaveName=ScopeData15
      Trq3 settings: SaveName=ScopeData16
      Trq4 settings: SaveName=ScopeData17
      Trq5 settings: SaveName=ScopeData18
      Trq6 settings: SaveName=ScopeData26
  Weld : mblibv1/Joints/Weld  LConnTagsString=__newl0  RConnTagsString=__newr0  UpdateFromCAD=on  NumSAPorts=0  CutJoint=off  MarkAsCut=off  Primitives=weld  PrimitiveProps=W$WORLD$[0.57735,0.57735,0.57735]$weld  DialogClass=JointBlock  WAxis=[0.57735,0.57735,0.57735]
  Out_R1 : Outport
  Out_R2 : Outport  Port=2
  Out_R3 : Outport  Port=3
  Out_R4 : Outport  Port=4
  Out_R5 : Outport  Port=5
  Out_R6 : Outport  Port=6
  Out_End : Outport  Port=7
  wires:
  In_R1/1 -> Actuator1/1, Trq1/1
  In_R2/1 -> Actuator2/1, Trq2/1
  JointSensor2/1(Out) -> Out_R2/1
  In_R3/1 -> Actuator3/1, Trq3/1
  JointSensor3/1(Out) -> Out_R3/1
  JointSensor4/1(Out) -> Out_R4/1
  In_R4/1 -> Actuator4/1, Trq4/1
  JointSensor5/1(Out) -> Out_R5/1
  In_R5/1 -> Actuator5/1, Trq5/1
  In_R6/1 -> Actuator6/1, Trq6/1
  " EndSensor"/1(Out) -> Out_End/1
  JointSensor1/1(Out) -> Out_R1/1
  JointSensor6/1(Out) -> Out_R6/1
  connections:
  " EndSensor"/LConn1 -- Body6/RConn1
  JointSensor6/LConn1 -- R6/RConn2
  Actuator6/RConn1 -- R6/LConn3
  Weld/LConn1 -- Ground/RConn1
  Actuator3/RConn1 -- R3/LConn3
  Init3/RConn1 -- R3/LConn2
  JointSensor3/LConn1 -- R3/RConn2
  Machine Environment/RConn1 -- Ground/LConn1
  R5/LConn1 -- Body4/RConn1
  R1/LConn1 -- Base/RConn1
  R6/RConn1 -- Body6/LConn1
  R5/RConn1 -- Body5/LConn1
  Body5/RConn1 -- R6/LConn1
  Body2/RConn1 -- R3/LConn1
  R2/RConn1 -- Body2/LConn1
  R2/LConn1 -- Body1/RConn1
  Weld/RConn1 -- Base/LConn1
  Actuator2/RConn1 -- R2/LConn3
  Init6/RConn1 -- R6/LConn2
  Body1/LConn1 -- R1/RConn1
  JointSensor2/LConn1 -- R2/RConn2
  Init2/RConn1 -- R2/LConn2
  R1/RConn2 -- JointSensor1/LConn1
  Actuator1/RConn1 -- R1/LConn3
  R1/LConn2 -- Init1/RConn1
  JointSensor5/LConn1 -- R5/RConn2
  R3/RConn1 -- Body3/LConn1
  Actuator5/RConn1 -- R5/LConn3
  Init5/RConn1 -- R5/LConn2
  R4/RConn1 -- Body4/LConn1
  R4/LConn1 -- Body3/RConn1
  Actuator4/RConn1 -- R4/LConn3
  Initi4/RConn1 -- R4/LConn2
  JointSensor4/LConn1 -- R4/RConn2

== system CtrPlatform/FbDisturb ==
  Constant : Constant  Value=0  SampleTime=Ts
  FbDisturbSelect : Constant  Value=FbDisturbSelect  SampleTime=Ts
  Gaussian Noise Generator : commnoisgen2/Gaussian Noise Generator  m=0  d=0.01  s=41  Ts=Ts  frameBased=off  sampPerFrame=1  orient=off  outDataType=double
  Multiport Switch : MultiPortSwitch  Inputs=2  zeroidx=off
  FbDisturb : Outport
  wires:
  Gaussian Noise Generator/1 -> Multiport Switch/2
  FbDisturbSelect/1 -> Multiport Switch/1
  Multiport Switch/1 -> FbDisturb/1
  Constant/1 -> Multiport Switch/3

== system CtrPlatform/Friction Torque ==
  Constant : Constant  Value=0  SampleTime=Ts
  Friction Torque : Subsystem
  FrictionSelect : Constant  Value=FrictionSelect  SampleTime=Ts
  Multiport Switch : MultiPortSwitch  Inputs=2  zeroidx=off
  Friction : Outport
  wires:
  Friction Torque/1(Friction Torque) -> Multiport Switch/2
  Constant/1 -> Multiport Switch/3
  Multiport Switch/1 -> Friction/1
  FrictionSelect/1 -> Multiport Switch/1

== system CtrPlatform/Signal Re-group ==
  In_R1 : Inport
  In_R2 : Inport  Port=2
  In_R3 : Inport  Port=3
  In_R4 : Inport  Port=4
  In_R5 : Inport  Port=5
  In_R6 : Inport  Port=6
  In_End : Inport  Port=7
  Demux : Demux  Outputs=3
  Re-group : Subsystem
  Re-group JntVelAcc : Subsystem
  Re-group_R1 : Subsystem
  Re-group_R2 : Subsystem
  Re-group_R3 : Subsystem
  Re-group_R4 : Subsystem
  Re-group_R5 : Subsystem
  Re-group_R6 : Subsystem
  Torque(Nm) : Outport
  End(mm/Deg) : Outport  Port=2
  JVAJVA(Deg) : Outport  Port=3
  Jnt(Deg) : Outport  Port=4
  tag scope: RobotEncAcc=global, RobotEncPos=global, RobotEncVel=global
  wires:
  In_R1/1 -> Re-group_R1/1(In_R1)
  In_R2/1 -> Re-group_R2/1(In_R2)
  In_R3/1 -> Re-group_R3/1(In_R3)
  In_R4/1 -> Re-group_R4/1(In_R4)
  In_R5/1 -> Re-group_R5/1(In_R5)
  In_R6/1 -> Re-group_R6/1(In_R6)
  Re-group/1(JntVelAcc) -> JVAJVA(Deg)/1, Re-group JntVelAcc/1(JntVelAcc)
  Re-group/2(Torque) -> Torque(Nm)/1
  In_End/1 -> End(mm/Deg)/1
  Re-group JntVelAcc/1(ReJntVelAcc) -> Demux/1
  Re-group_R1/1(JntVelAcc_R1) -> Re-group/1(JntVelAcc_R1)
  Re-group_R1/2(Torque_R1) -> Re-group/2(Torque_R1)
  Re-group_R2/1(JntVelAcc_R2) -> Re-group/3(JntVelAcc_R2)
  Re-group_R2/2(Torque_R2) -> Re-group/4(Torque_R2)
  Re-group_R3/1(JntVelAcc_R3) -> Re-group/5(JntVelAcc_R3)
  Re-group_R3/2(Torque_R3) -> Re-group/6(Torque_R3)
  Re-group_R4/1(JntVelAcc_R4) -> Re-group/7(JntVelAcc_R4)
  Re-group_R4/2(Torque_R4) -> Re-group/8(Torque_R4)
  Re-group_R5/1(JntVelAcc_R5) -> Re-group/9(JntVelAcc_R5)
  Re-group_R5/2(Torque_R5) -> Re-group/10(Torque_R5)
  Re-group_R6/1(JntVelAcc_R6) -> Re-group/11(JntVelAcc_R6)
  Re-group_R6/2(Torque_R6) -> Re-group/12(Torque_R6)
  Demux/3 -> [RobotEncAcc]
  Demux/2 -> [RobotEncVel]
  Demux/1 -> [RobotEncPos], Jnt(Deg)/1

== system CtrPlatform/Trajectory Generator ==
  Circle in Descartes Space : Subsystem
  Demux : Demux  Outputs=3
  End Switch : MultiPortSwitch  zeroidx=off
  JJVVAA Switch : MultiPortSwitch  zeroidx=off
  JVA Switch : MultiPortSwitch  zeroidx=off
  Line in Joint Space : Subsystem
  Still : Subsystem
  Switch : Constant  Value=TrajSwitch  SampleTime=Ts_Dyn
  Ref_Jnt : Outport
  Ref_End : Outport  Port=2
  Ref_JVAJVA : Outport  Port=3
  tag scope: RobotProfileAcc=global, RobotProfilePos=global, RobotProfileVel=global
  wires:
  Switch/1 -> JJVVAA Switch/1, JVA Switch/1, End Switch/1
  Still/1(Ref_JJVVAA) -> JJVVAA Switch/3
  Circle in Descartes Space/2(RefEnd) -> End Switch/2
  Still/2(RefEnd) -> End Switch/3
  Line in Joint Space/2(RefEnd) -> End Switch/4
  Circle in Descartes Space/3(Ref_JVAJVA) -> JVA Switch/2
  Still/3(Ref_JVAJVA) -> JVA Switch/3
  Line in Joint Space/3(Ref_JVAJVA) -> JVA Switch/4
  End Switch/1 -> Ref_End/1
  JVA Switch/1 -> Ref_JVAJVA/1
  Demux/1 -> [RobotProfilePos], Ref_Jnt/1
  Demux/2 -> [RobotProfileVel]
  Demux/3 -> [RobotProfileAcc]
  Circle in Descartes Space/1(Ref_JJVVAA) -> JJVVAA Switch/2
  Line in Joint Space/1(Ref_JJVVAA) -> JJVVAA Switch/4
  JJVVAA Switch/1 -> Demux/1

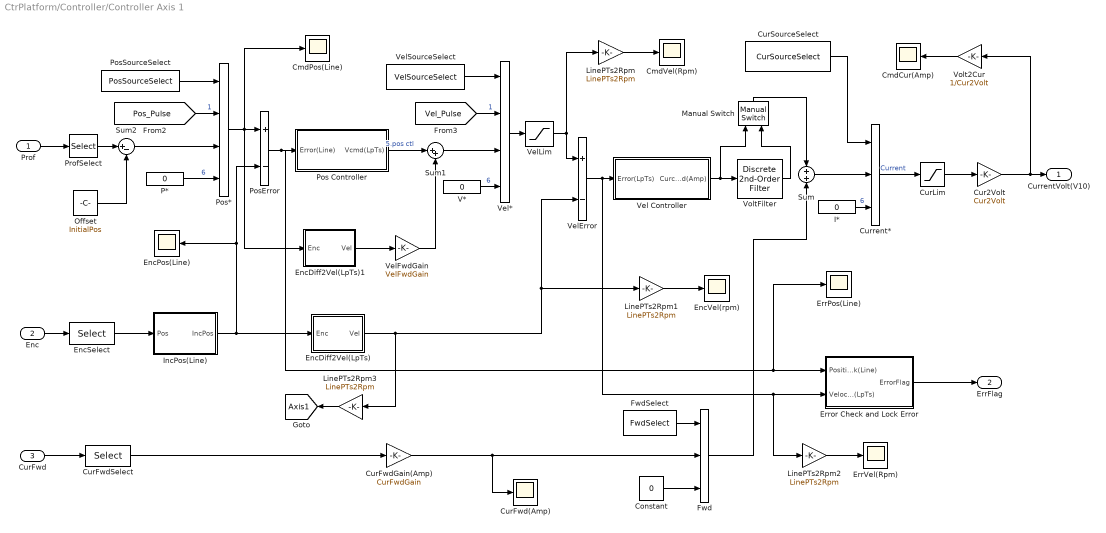
== system CtrPlatform/Controller/Controller Axis 1 ==
  Prof : Inport
  Enc : Inport  Port=2
  CurFwd : Inport  Port=3
  CmdCur(Amp) : Scope
      settings: SaveName=ScopeData42
  CmdPos(Line) : Scope
      settings: SaveName=ScopeData40
  CmdVel(Rpm) : Scope
      settings: SaveName=ScopeData39
  Constant : Constant  Value=0
  Cur2Volt : Gain  Gain=Cur2Volt  SampleTime=Ts
  CurFwd(Amp) : Scope
      settings: TimeRange=5  YMin=-600  YMax=600  SaveName=ScopeData14
  CurFwdGain(Amp) : Gain  Gain=CurFwdGain
  CurFwdSelect : Selector  InputPortWidth=6  IndexOptions=Index vector (dialog)  Indices=AxisNO  OutputSizes=1
  CurLim : Saturate  UpperLimit=CurLimit  LowerLimit=-CurLimit  SampleTime=Ts
  CurSourceSelect : Constant  Value=CurSourceSelect  SampleTime=Ts
  Current* : MultiPortSwitch  Inputs=2  zeroidx=off
  EncDiff2Vel(LpTs) : Subsystem
  EncDiff2Vel(LpTs)1 : Subsystem
  EncPos(Line) : Scope
      settings: SaveName=ScopeData41
  "EncSelect " : Selector  InputPortWidth=6  IndexOptions=Index vector (dialog)  Indices=AxisNO  OutputSizes=1
  EncVel(rpm) : Scope
      settings: SaveName=ScopeData43
  ErrPos(Line) : Scope
      settings: SaveName=ScopeData44
  ErrVel(Rpm) : Scope
      settings: SaveName=ScopeData45
  Error Check and Lock Error : Subsystem
  Fwd : MultiPortSwitch  Inputs=2  zeroidx=off
  FwdSelect : Constant  Value=FwdSelect  SampleTime=Ts
  I* : Constant  Value=0  SampleTime=Ts
  IncPos(Line) : Subsystem
  LinePTs2Rpm{,1..3} (4 alike) : Gain  Gain=LinePTs2Rpm
  Manual Switch : simulink/Signal Routing/Manual Switch  sw=1  action=0  varsize=off
  Offset : Constant  Value=InitialPos  SampleTime=-1
  P* : Constant  Value=0  SampleTime=Ts
  Pos Controller : Subsystem  mask{Kp=Kpp, Ki=Kpi, Kd=Kpd, Ts=Ts}
      mask prompts: Ts "Sample Time"
  Pos* : MultiPortSwitch  zeroidx=off
  PosError : Sum  Inputs=+-
  PosSourceSelect : Constant  Value=PosSourceSelect  SampleTime=Ts
  ProfSelect : Selector  InputPortWidth=6  IndexOptions=Index vector (dialog)  Indices=AxisNO  OutputSizes=1
  Sum : Sum  Inputs=+|+
  Sum1 : Sum  Inputs=|++
  Sum2 : Sum  Inputs=|+-
  V* : Constant  Value=0  SampleTime=Ts
  Vel Controller : Subsystem  mask{Kp=Kvp, Ki=Kvi, Kd=Kvd, Ts=Ts}
      mask prompts: Ts "Sample Time"
  Vel* : MultiPortSwitch  zeroidx=off
  VelError : Sum  Inputs=+-
  VelFwdGain : Gain  Gain=VelFwdGain
  VelLim : Saturate  UpperLimit=VelLimit  LowerLimit=-VelLimit  SampleTime=Ts
  VelSourceSelect : Constant  Value=VelSourceSelect  SampleTime=Ts
  Volt2Cur : Gain  Gain=1/Cur2Volt  SampleTime=Ts
  VoltFilter : powerlib_extras/Discrete  Control Blocks/Discrete  2nd-Order Filter  FilterType=Lowpass  Fo=200  Zeta=0.707  Ts=Ts  Initialize=off  Vac_Init=[0.8 -25 60]  Vdc_Init=-0.4  PlotResponse=off  param1=[1 500 1]
  CurrentVolt(V10) : Outport
  ErrFlag : Outport  Port=2
  tag scope: Axis1=global
  wires:
  I*/1 -> Current*/3  "6"
  EncDiff2Vel(LpTs)1/1(Vel) -> VelFwdGain/1
  VelFwdGain/1 -> Sum1/2
  Volt2Cur/1 -> CmdCur(Amp)/1
  LinePTs2Rpm2/1 -> ErrVel(Rpm)/1
  LinePTs2Rpm1/1 -> EncVel(rpm)/1
  LinePTs2Rpm/1 -> CmdVel(Rpm)/1
  Cur2Volt/1 -> Volt2Cur/1, CurrentVolt(V10)/1
  CurLim/1 -> Cur2Volt/1
  VelLim/1 -> LinePTs2Rpm/1, VelError/1
  Sum1/1 -> Vel*/3
  Pos Controller/1(Vcmd(LpTs)) -> Sum1/1  "5.pos ctl"
  CurFwdGain(Amp)/1 -> CurFwd(Amp)/1, Fwd/2
  CurFwdSelect/1 -> CurFwdGain(Amp)/1
  CurFwd/1 -> CurFwdSelect/1
  V*/1 -> Vel*/4  "6"
  [Pos_Pulse] -> Pos*/2  "1"
  P*/1 -> Pos*/4  "6"
  [Vel_Pulse] -> Vel*/2  "1"
  Pos*/1 -> PosError/1, EncDiff2Vel(LpTs)1/1(Enc), CmdPos(Line)/1
  PosSourceSelect/1 -> Pos*/1
  Vel*/1 -> VelLim/1
  "EncSelect "/1 -> IncPos(Line)/1(Pos)
  Enc/1 -> "EncSelect "/1
  Prof/1 -> ProfSelect/1
  EncDiff2Vel(LpTs)/1(Vel) -> LinePTs2Rpm3/1, VelError/2, LinePTs2Rpm1/1
  VelError/1 -> LinePTs2Rpm2/1, Error Check and Lock Error/2(VelocityCheck(LpTs)), Vel Controller/1(Error(LpTs))
  VelSourceSelect/1 -> Vel*/1
  CurSourceSelect/1 -> Current*/1
  PosError/1 -> ErrPos(Line)/1, Error Check and Lock Error/1(PositionCheck(Line)), Pos Controller/1(Error(Line))
  Current*/1 -> CurLim/1  "Current"
  Error Check and Lock Error/1(ErrorFlag) -> ErrFlag/1
  IncPos(Line)/1(IncPos) -> EncPos(Line)/1, PosError/2, EncDiff2Vel(LpTs)/1(Enc)
  ProfSelect/1 -> Sum2/1
  Sum2/1 -> Pos*/3
  Offset/1 -> Sum2/2
  Vel Controller/1(Curcmd(Amp)) -> VoltFilter/1, Manual Switch/1
  VoltFilter/1 -> Manual Switch/2
  Manual Switch/1 -> Sum/1
  Sum/1 -> Current*/2
  Fwd/1 -> Sum/2
  Constant/1 -> Fwd/3
  FwdSelect/1 -> Fwd/1
  LinePTs2Rpm3/1 -> [Axis1]

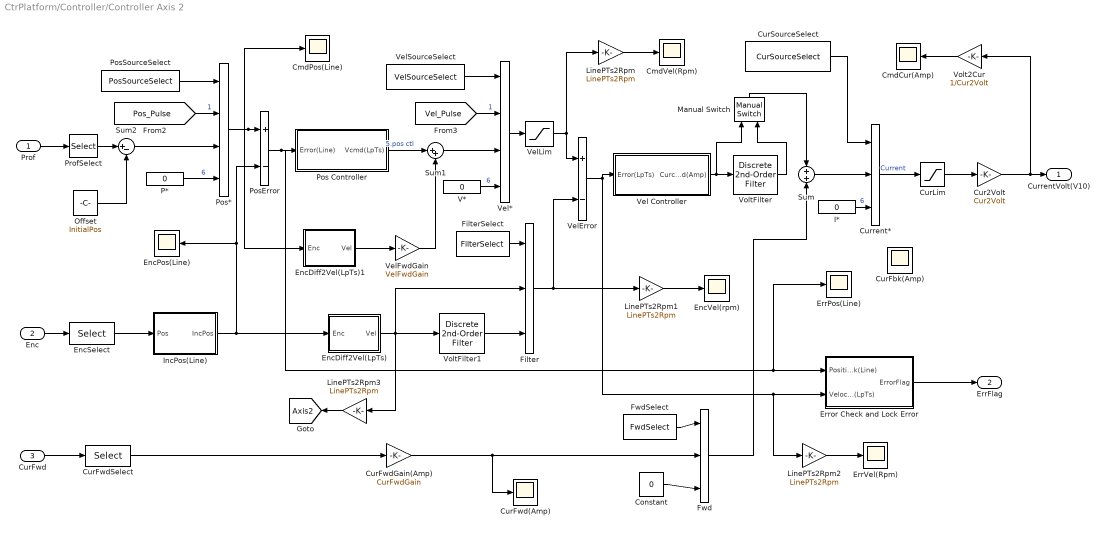
== system CtrPlatform/Controller/Controller Axis 2 ==
  Prof : Inport
  Enc : Inport  Port=2
  CurFwd : Inport  Port=3
  CmdCur(Amp) : Scope
      settings: SaveName=ScopeData42
  CmdPos(Line) : Scope
      settings: SaveName=ScopeData40
  CmdVel(Rpm) : Scope
      settings: SaveName=ScopeData39
  Constant : Constant  Value=0
  Cur2Volt : Gain  Gain=Cur2Volt  SampleTime=Ts
  CurFbk(Amp) : Scope
      settings: SaveName=ScopeData27
  CurFwd(Amp) : Scope
      settings: TimeRange=5  YMin=-600  YMax=600  SaveName=ScopeData14
  CurFwdGain(Amp) : Gain  Gain=CurFwdGain
  CurFwdSelect : Selector  InputPortWidth=6  IndexOptions=Index vector (dialog)  Indices=AxisNO  OutputSizes=1
  CurLim : Saturate  UpperLimit=CurLimit  LowerLimit=-CurLimit  SampleTime=Ts
  CurSourceSelect : Constant  Value=CurSourceSelect  SampleTime=Ts
  Current* : MultiPortSwitch  Inputs=2  zeroidx=off
  EncDiff2Vel(LpTs) : Subsystem
  EncDiff2Vel(LpTs)1 : Subsystem
  EncPos(Line) : Scope
      settings: SaveName=ScopeData41
  "EncSelect " : Selector  InputPortWidth=6  IndexOptions=Index vector (dialog)  Indices=AxisNO  OutputSizes=1
  EncVel(rpm) : Scope
      settings: SaveName=ScopeData43
  ErrPos(Line) : Scope
      settings: SaveName=ScopeData44
  ErrVel(Rpm) : Scope
      settings: SaveName=ScopeData45
  Error Check and Lock Error : Subsystem
  Filter : MultiPortSwitch  Inputs=2  zeroidx=off
  FilterSelect : Constant  Value=FilterSelect  SampleTime=Ts
  Fwd : MultiPortSwitch  Inputs=2  zeroidx=off
  FwdSelect : Constant  Value=FwdSelect  SampleTime=Ts
  I* : Constant  Value=0  SampleTime=Ts
  IncPos(Line) : Subsystem
  LinePTs2Rpm{,1..3} (4 alike) : Gain  Gain=LinePTs2Rpm
  Manual Switch : simulink/Signal Routing/Manual Switch  sw=1  action=0  varsize=off
  Offset : Constant  Value=InitialPos  SampleTime=-1
  P* : Constant  Value=0  SampleTime=Ts
  Pos Controller : Subsystem  mask{Kp=Kpp, Ki=Kpi, Kd=Kpd, Ts=Ts}
      mask prompts: Ts "Sample Time"
  Pos* : MultiPortSwitch  zeroidx=off
  PosError : Sum  Inputs=+-
  PosSourceSelect : Constant  Value=PosSourceSelect  SampleTime=Ts
  ProfSelect : Selector  InputPortWidth=6  IndexOptions=Index vector (dialog)  Indices=AxisNO  OutputSizes=1
  Sum : Sum  Inputs=+|+
  Sum1 : Sum  Inputs=|++
  Sum2 : Sum  Inputs=|+-
  V* : Constant  Value=0  SampleTime=Ts
  Vel Controller : Subsystem  mask{Kp=Kvp, Ki=Kvi, Kd=Kvd, Ts=Ts}
      mask prompts: Ts "Sample Time"
  Vel* : MultiPortSwitch  zeroidx=off
  VelError : Sum  Inputs=+-
  VelFwdGain : Gain  Gain=VelFwdGain
  VelLim : Saturate  UpperLimit=VelLimit  LowerLimit=-VelLimit  SampleTime=Ts
  VelSourceSelect : Constant  Value=VelSourceSelect  SampleTime=Ts
  Volt2Cur : Gain  Gain=1/Cur2Volt  SampleTime=Ts
  VoltFilter : powerlib_extras/Discrete  Control Blocks/Discrete  2nd-Order Filter  FilterType=Lowpass  Fo=200  Zeta=0.707  Ts=Ts  Initialize=off  Vac_Init=[0.8 -25 60]  Vdc_Init=-0.4  PlotResponse=off  param1=[1 500 1]
  VoltFilter1 : powerlib_extras/Discrete  Control Blocks/Discrete  2nd-Order Filter  FilterType=Lowpass  Fo=200  Zeta=0.707  Ts=Ts  Initialize=off  Vac_Init=[0.8 -25 60]  Vdc_Init=-0.4  PlotResponse=off  param1=[1 500 1]
  CurrentVolt(V10) : Outport
  ErrFlag : Outport  Port=2
  tag scope: Axis2=global
  wires:
  I*/1 -> Current*/3  "6"
  EncDiff2Vel(LpTs)1/1(Vel) -> VelFwdGain/1
  VelFwdGain/1 -> Sum1/2
  Volt2Cur/1 -> CmdCur(Amp)/1
  LinePTs2Rpm2/1 -> ErrVel(Rpm)/1
  LinePTs2Rpm1/1 -> EncVel(rpm)/1
  LinePTs2Rpm/1 -> CmdVel(Rpm)/1
  Cur2Volt/1 -> Volt2Cur/1, CurrentVolt(V10)/1
  CurLim/1 -> Cur2Volt/1
  VelLim/1 -> LinePTs2Rpm/1, VelError/1
  Sum1/1 -> Vel*/3
  Pos Controller/1(Vcmd(LpTs)) -> Sum1/1  "5.pos ctl"
  CurFwdGain(Amp)/1 -> CurFwd(Amp)/1, Fwd/2
  CurFwdSelect/1 -> CurFwdGain(Amp)/1
  CurFwd/1 -> CurFwdSelect/1
  V*/1 -> Vel*/4  "6"
  [Pos_Pulse] -> Pos*/2  "1"
  P*/1 -> Pos*/4  "6"
  [Vel_Pulse] -> Vel*/2  "1"
  Pos*/1 -> PosError/1, EncDiff2Vel(LpTs)1/1(Enc), CmdPos(Line)/1
  PosSourceSelect/1 -> Pos*/1
  Vel*/1 -> VelLim/1
  "EncSelect "/1 -> IncPos(Line)/1(Pos)
  Enc/1 -> "EncSelect "/1
  Prof/1 -> ProfSelect/1
  EncDiff2Vel(LpTs)/1(Vel) -> VoltFilter1/1, Filter/2, LinePTs2Rpm3/1
  VelError/1 -> LinePTs2Rpm2/1, Error Check and Lock Error/2(VelocityCheck(LpTs)), Vel Controller/1(Error(LpTs))
  VelSourceSelect/1 -> Vel*/1
  CurSourceSelect/1 -> Current*/1
  PosError/1 -> ErrPos(Line)/1, Error Check and Lock Error/1(PositionCheck(Line)), Pos Controller/1(Error(Line))
  Current*/1 -> CurLim/1  "Current"
  Error Check and Lock Error/1(ErrorFlag) -> ErrFlag/1
  IncPos(Line)/1(IncPos) -> EncPos(Line)/1, PosError/2, EncDiff2Vel(LpTs)/1(Enc)
  ProfSelect/1 -> Sum2/1
  Sum2/1 -> Pos*/3
  Offset/1 -> Sum2/2
  Vel Controller/1(Curcmd(Amp)) -> VoltFilter/1, Manual Switch/1
  VoltFilter/1 -> Manual Switch/2
  Manual Switch/1 -> Sum/1
  Sum/1 -> Current*/2
  Fwd/1 -> Sum/2
  VoltFilter1/1 -> Filter/3
  Filter/1 -> VelError/2, LinePTs2Rpm1/1
  FilterSelect/1 -> Filter/1
  Constant/1 -> Fwd/3
  FwdSelect/1 -> Fwd/1
  LinePTs2Rpm3/1 -> [Axis2]
